simulink model "Obs_ex_do"  (R2018a)
settings: Solver=VariableStepAuto  StartTime=0.0  StopTime=10.0  RelTol=1e-3
undefined symbols (not defined in the file): A, B, C, D, F, G, L, simSwitch, Ts, x0, x0_h
settings Model: Creator=pala  LastModifiedBy=pala
settings DataIOCC: FinalStateName=xF_do  SaveFinalState=on  SaveFormat=StructureWithTime  SaveState=on  SignalLogging=off  DSMLogging=off  StateSaveName=x_do  TimeSaveName=t_do  OutputSaveName=y_do

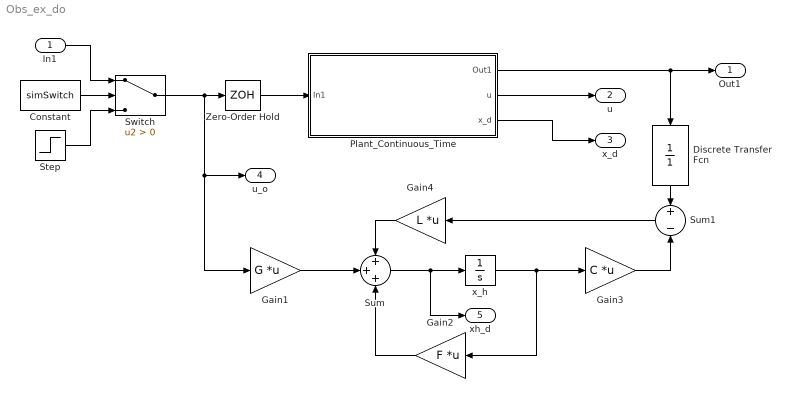
== system Obs_ex_do ==
  In1 : Inport
  Constant : Constant  Value=simSwitch
  Discrete Transfer Fcn : DiscreteTransferFcn  Denominator=[1 ]  SampleTime=Ts
  Gain1 : Gain  Gain=G  Multiplication=Matrix(K*u)
  Gain2 : Gain  Gain=F  Multiplication=Matrix(K*u)
  Gain3 : Gain  Gain=C  Multiplication=Matrix(K*u)
  Gain4 : Gain  Gain=L  Multiplication=Matrix(K*u)
  "Plant_Continuous_Time " : Subsystem
  Step : Step  SampleTime=0
  Sum : Sum  Inputs=+++
  Sum1 : Sum  Inputs=+-
  Switch : Switch  Criteria=u2 > Threshold
  Zero-Order Hold : ZeroOrderHold  SampleTime=Ts
  x_h : Integrator  Priority=2  InitialCondition=x0_h
  Out1 : Outport
  u : Outport  Port=2
  x_d : Outport  Port=3
  u_o : Outport  Port=4
  xh_d : Outport  Port=5
  wires:
  In1/1 -> Switch/1
  Step/1 -> Switch/3
  Constant/1 -> Switch/2
  Gain1/1 -> Sum/2
  Sum/1 -> xh_d/1, x_h/1
  Gain2/1 -> Sum/3
  x_h/1 -> Gain3/1, Gain2/1
  Gain4/1 -> Sum/1
  Sum1/1 -> Gain4/1
  Gain3/1 -> Sum1/2
  Switch/1 -> Zero-Order Hold/1, u_o/1, Gain1/1
  "Plant_Continuous_Time "/1(Out1) -> Discrete Transfer Fcn/1, Out1/1
  "Plant_Continuous_Time "/2(u) -> u/1
  "Plant_Continuous_Time "/3(x_d) -> x_d/1
  Zero-Order Hold/1 -> "Plant_Continuous_Time "/1(In1)
  Discrete Transfer Fcn/1 -> Sum1/1

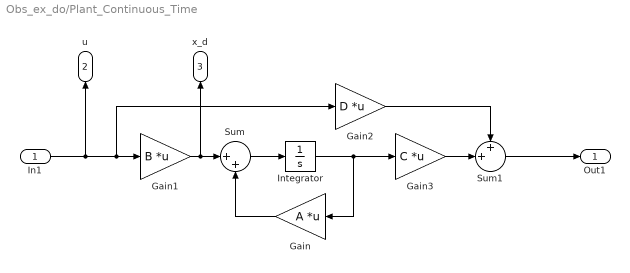
== system Obs_ex_do/Plant_Continuous_Time  ==
  In1 : Inport
  Gain : Gain  Gain=A  Multiplication=Matrix(K*u)
  Gain1 : Gain  Gain=B  Multiplication=Matrix(K*u)
  Gain2 : Gain  Gain=D  Multiplication=Matrix(K*u)
  Gain3 : Gain  Gain=C  Multiplication=Matrix(K*u)
  Integrator : Integrator  Priority=1  InitialCondition=x0
  Sum : Sum  Inputs=|++
  Sum1 : Sum  Inputs=++|
  Out1 : Outport
  u : Outport  Port=2
  x_d : Outport  Port=3
  wires:
  Integrator/1 -> Gain3/1, Gain/1
  Gain1/1 -> x_d/1, Sum/1
  Gain2/1 -> Sum1/1
  Gain/1 -> Sum/2
  Sum/1 -> Integrator/1
  Gain3/1 -> Sum1/2
  Sum1/1 -> Out1/1
  In1/1 -> u/1, Gain2/1, Gain1/1
